simulink library "nonlinearPlnt_ul"  (R2018a)
settings: Solver=VariableStepAuto  StartTime=0.0  StopTime=10.0  RelTol=1e-3
values from neighbouring files (symbols this model uses):
  initialHeading_deg = (180/pi)*atan2(v(2),v(1))    [nonlinearPlnt_ul_init.m]
  initialSpeed_mPs = 5    [nonlinearPlnt_ul_init.m]
  initialXPosition_m = 0    [nonlinearPlnt_ul_init.m]
  initialYPosition_m = 0    [nonlinearPlnt_ul_init.m]
libraries: stateEquations_ul x1
settings Model: Creator=mcobb  LastModifiedBy=mcobb

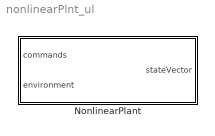
== system nonlinearPlnt_ul ==
  NonlinearPlant : Subsystem

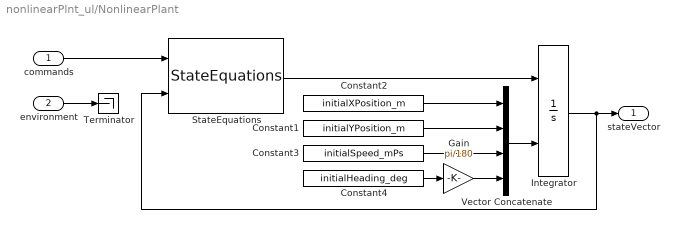
== system nonlinearPlnt_ul/NonlinearPlant ==
  commands : Inport
  environment : Inport  Port=2
  Constant1 : Constant  Value=initialYPosition_m
  Constant2 : Constant  Value=initialXPosition_m
  Constant3 : Constant  Value=initialSpeed_mPs
  Constant4 : Constant  Value=initialHeading_deg
  Gain : Gain  Gain=pi/180
  Integrator : Integrator  InitialConditionSource=external
  StateEquations : stateEquations_ul/StateEquations
  Terminator : Terminator
  Vector Concatenate : Concatenate  NumInputs=4
  stateVector : Outport
  wires:
  StateEquations/1 -> Integrator/1
  Vector Concatenate/1 -> Integrator/2
  Constant2/1 -> Vector Concatenate/1
  Constant1/1 -> Vector Concatenate/2
  Constant3/1 -> Vector Concatenate/3
  Constant4/1 -> Gain/1
  Gain/1 -> Vector Concatenate/4
  Integrator/1 -> StateEquations/2, stateVector/1
  commands/1 -> StateEquations/1
  environment/1 -> Terminator/1
